simulink model "Model01"  (R2017b)
settings: Solver=VariableStepAuto  StartTime=0.0  StopTime=20  RelTol=1e-3
settings Model: Creator=jim  LastModifiedBy=jim

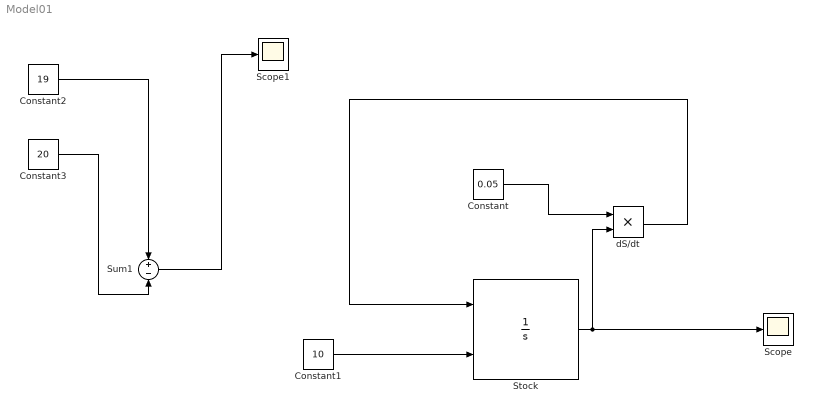
== system Model01 ==
  Constant : Constant  Value=0.05
  Constant1 : Constant  Value=10
  Constant2 : Constant  Value=19
  Constant3 : Constant  Value=20
  Scope : Scope
  Scope1 : Scope
  Stock : Integrator  InitialConditionSource=external
  Sum1 : Sum  Inputs=+-
  dS/dt : Product
  wires:
  Constant1/1 -> Stock/2
  Stock/1 -> dS/dt/2, Scope/1
  dS/dt/1 -> Stock/1
  Constant/1 -> dS/dt/1
  Constant2/1 -> Sum1/1
  Constant3/1 -> Sum1/2
  Sum1/1 -> Scope1/1
